simulink model "reshapedevel"  (Simulink 7.4)
settings: Solver=ode45  StartTime=0.0  StopTime=800  RelTol=1e-3
libraries: xbsIndex_r4 x41, casper_library_misc x3
settings Model: Creator=gjones  LastModifiedBy=gjones

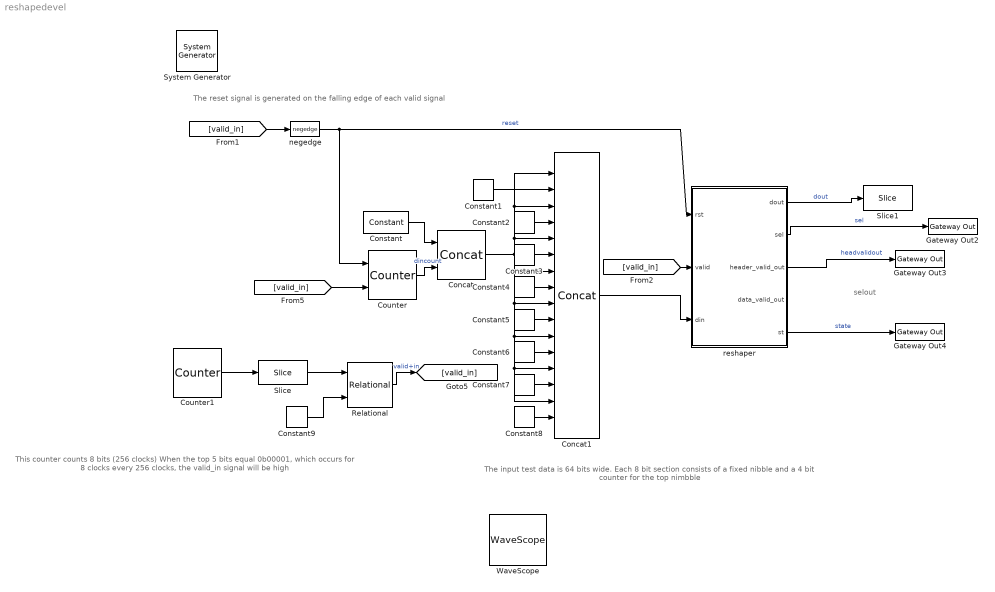
== system reshapedevel ==
  note: selout
  note: This counter counts 8 bits (256 clocks)
      | When the top 5 bits equal 0b00001, which occurs for 8
      | clocks every 256 clocks, the valid_in signal will be high
  note: The reset signal is generated on the falling edge of each valid signal
  note: The input test data is 64 bits wide. Each 8 bit section consists of a fixed nibble and
      |  a 4 bit counter for the top nimbble
  " System Generator" : xbsIndex_r4/ System Generator  Tag=genX  SystemSampleTime=-1  xilinxfamily=Virtex6  part=xc6vsx315t  speed=-3  package=ff1156  synthesis_tool=XST  clock_wrapper=Clock Enables  directory=./netlist  testbench=off  simulink_period=1  sysclk_period=10  dcm_input_clock_period=10  incr_netlist=off  trim_vbits=Everywhere in SubSystem  dbl_ovrd=According to Block Masks  core_generation=According to Block Masks  run_coregen=off  deprecated_control=off  eval_field=0  block_type=sysgen
      settings: block_version=11.4
  Concat : xbsIndex_r4/Concat  num_inputs=2  dbl_ovrd=off  block_type=concat
  Concat1 : xbsIndex_r4/Concat  num_inputs=16  dbl_ovrd=off  block_type=concat
  Constant : xbsIndex_r4/Constant  arith_type=Unsigned  const=0  n_bits=1  bin_pt=0  explicit_period=on  period=1  equ=P=C  opselect=C  inp2=PCIN>>17  opr=+  inp1=P  carry=CIN  dbl_ovrd=off  block_type=constant
      settings: block_version=11.4
  Constant1 : xbsIndex_r4/Constant  arith_type=Unsigned  const=0  n_bits=4  bin_pt=0  explicit_period=on  period=1  equ=P=C  opselect=C  inp2=PCIN>>17  opr=+  inp1=P  carry=CIN  dbl_ovrd=off  block_type=constant
      settings: block_version=11.4
  Constant2 : xbsIndex_r4/Constant  arith_type=Unsigned  const=1  n_bits=4  bin_pt=0  explicit_period=on  period=1  equ=P=C  opselect=C  inp2=PCIN>>17  opr=+  inp1=P  carry=CIN  dbl_ovrd=off  block_type=constant
      settings: block_version=11.4
  Constant3 : xbsIndex_r4/Constant  arith_type=Unsigned  const=2  n_bits=4  bin_pt=0  explicit_period=on  period=1  equ=P=C  opselect=C  inp2=PCIN>>17  opr=+  inp1=P  carry=CIN  dbl_ovrd=off  block_type=constant
      settings: block_version=11.4
  Constant4 : xbsIndex_r4/Constant  arith_type=Unsigned  const=3  n_bits=4  bin_pt=0  explicit_period=on  period=1  equ=P=C  opselect=C  inp2=PCIN>>17  opr=+  inp1=P  carry=CIN  dbl_ovrd=off  block_type=constant
      settings: block_version=11.4
  Constant5 : xbsIndex_r4/Constant  arith_type=Unsigned  const=4  n_bits=4  bin_pt=0  explicit_period=on  period=1  equ=P=C  opselect=C  inp2=PCIN>>17  opr=+  inp1=P  carry=CIN  dbl_ovrd=off  block_type=constant
      settings: block_version=11.4
  Constant6 : xbsIndex_r4/Constant  arith_type=Unsigned  const=5  n_bits=4  bin_pt=0  explicit_period=on  period=1  equ=P=C  opselect=C  inp2=PCIN>>17  opr=+  inp1=P  carry=CIN  dbl_ovrd=off  block_type=constant
      settings: block_version=11.4
  Constant7 : xbsIndex_r4/Constant  arith_type=Unsigned  const=6  n_bits=4  bin_pt=0  explicit_period=on  period=1  equ=P=C  opselect=C  inp2=PCIN>>17  opr=+  inp1=P  carry=CIN  dbl_ovrd=off  block_type=constant
      settings: block_version=11.4
  Constant8 : xbsIndex_r4/Constant  arith_type=Unsigned  const=7  n_bits=4  bin_pt=0  explicit_period=on  period=1  equ=P=C  opselect=C  inp2=PCIN>>17  opr=+  inp1=P  carry=CIN  dbl_ovrd=off  block_type=constant
      settings: block_version=11.4
  Constant9 : xbsIndex_r4/Constant  arith_type=Unsigned  const=1  n_bits=4  bin_pt=0  explicit_period=on  period=1  equ=P=C  opselect=C  inp2=PCIN>>17  opr=+  inp1=P  carry=CIN  dbl_ovrd=off  block_type=constant
      settings: block_version=11.4
  Counter : xbsIndex_r4/Counter  cnt_type=Free Running  cnt_to=Inf  operation=Up  start_count=0  cnt_by_val=1  arith_type=Unsigned  n_bits=3  bin_pt=0  load_pin=off  rst=on  en=on  explicit_period=on  period=1  dbl_ovrd=off  use_behavioral_HDL=off  implementation=Fabric  block_type=counter
      settings: block_version=11.4
  Counter1 : xbsIndex_r4/Counter  cnt_type=Free Running  cnt_to=Inf  operation=Up  start_count=0  cnt_by_val=1  arith_type=Unsigned  n_bits=8  bin_pt=0  load_pin=off  rst=off  en=off  explicit_period=on  period=1  dbl_ovrd=off  use_behavioral_HDL=off  implementation=Fabric  block_type=counter
      settings: block_version=11.4
  Gateway Out2 : xbsIndex_r4/Gateway Out  hdl_port=on  timing_constraint=None  locs_specified=off  LOCs={}  block_type=gatewayout
      settings: infoedit="Gateway out block.  Converts Xilinx fixed point inputs into ouputs of type Simulink integer, double, or fixed point.<br><br>Hardware notes:  In hardware these blocks become top level output ports or are discarded, depending on how they are configured."  block_version=11.4
  Gateway Out3 : xbsIndex_r4/Gateway Out  hdl_port=on  timing_constraint=None  locs_specified=off  LOCs={}  block_type=gatewayout
      settings: infoedit="Gateway out block.  Converts Xilinx fixed point inputs into ouputs of type Simulink integer, double, or fixed point.<br><br>Hardware notes:  In hardware these blocks become top level output ports or are discarded, depending on how they are configured."  block_version=11.4
  Gateway Out4 : xbsIndex_r4/Gateway Out  hdl_port=on  timing_constraint=None  locs_specified=off  LOCs={}  block_type=gatewayout
      settings: infoedit="Gateway out block.  Converts Xilinx fixed point inputs into ouputs of type Simulink integer, double, or fixed point.<br><br>Hardware notes:  In hardware these blocks become top level output ports or are discarded, depending on how they are configured."  block_version=11.4
  Relational : xbsIndex_r4/Relational  mode=a=b  en=off  latency=0  dbl_ovrd=off  block_type=relational
  Slice : xbsIndex_r4/Slice  nbits=5  boolean_output=off  mode=Upper Bit Location + Width  bit1=0  base1=MSB of Input  bit0=0  base0=LSB of Input  dbl_ovrd=off  block_type=slice
  Slice1 : xbsIndex_r4/Slice  nbits=4  boolean_output=off  mode=Upper Bit Location + Width  bit1=0  base1=MSB of Input  bit0=0  base0=LSB of Input  dbl_ovrd=off  block_type=slice
  WaveScope : xbsIndex_r4/WaveScope  block_type=wavescope
      settings: block_version=11.4
  negedge : casper_library_misc/negedge  Tag=Rising Edge Detector  SystemSampleTime=-1
  reshaper : Subsystem  mask{inwid=64, inlen=8, outwid=8, outchunk=16, headlen=11}
      mask prompts: inwid "Input Width (bits)"; inlen "Input Length (clocks)"; outwid "Output Width (bits)"; outchunk "Output Chunk Length (clocks)"; headlen "Header Length"
      mask help:
      | This block takes wide input data and reshapes it to a narrower (or the same)
      | bit width, and breaks it into packets, between which a header can be inserted.
      | Each input data frame must be proceeded by a reset pulse. The input data can be
      | disjoint, with a pulsed valid signal. When the reset signal is pulsed, the previous data
      | frame will be read out. Therefore the number of clocks to read out the header and
      | data must be greater than the number of clocks between two frames (rst signals).
      |
      | The sel signal can be used to drive the select input of a mux which muxes between
      | the data stream (dout) and the indicated number of header words. The header_valid_out
      | signal goes high for each word of the header. dout should be connected to input
      | 0 of the mux. The data_valid_out goes high for each output data value. The st output
      | is for debug access to the internal state machine state.
      mask init:
      | l2inlen = ceil(log2(inlen))
      | l2outchunk = ceil(log2(outchunk))
      | outlen = inlen*(inwid/outwid)
      | nchunk = outlen/outchunk
      | l2headlen = ceil(log2(headlen))
      | l2outlen = ceil(log2(outlen))
  wires:
  Constant/1 -> Concat/1
  Counter/1 -> Concat/2  "dincount"
  Concat/1 -> Concat1/1, Concat1/3, Concat1/5, Concat1/7, Concat1/9, Concat1/11, Concat1/13, Concat1/15
  Constant1/1 -> Concat1/2
  Constant2/1 -> Concat1/4
  Constant3/1 -> Concat1/6
  Constant4/1 -> Concat1/8
  Constant5/1 -> Concat1/10
  Constant6/1 -> Concat1/12
  Constant7/1 -> Concat1/14
  Constant8/1 -> Concat1/16
  Concat1/1 -> reshaper/3(din)
  negedge/1 -> Counter/1, reshaper/1(rst)  "reset"
  Counter1/1 -> Slice/1
  Slice/1 -> Relational/1
  Constant9/1 -> Relational/2
  Relational/1 -> [valid_in]  "valid+in"
  reshaper/1(dout) -> Slice1/1  "dout"
  reshaper/2(sel) -> Gateway Out2/1  "sel"
  reshaper/3(header_valid_out) -> Gateway Out3/1  "headvalidout"
  reshaper/5(st) -> Gateway Out4/1  "state"
  [valid_in] -> Counter/2
  [valid_in] -> negedge/1
  [valid_in] -> reshaper/2(valid)

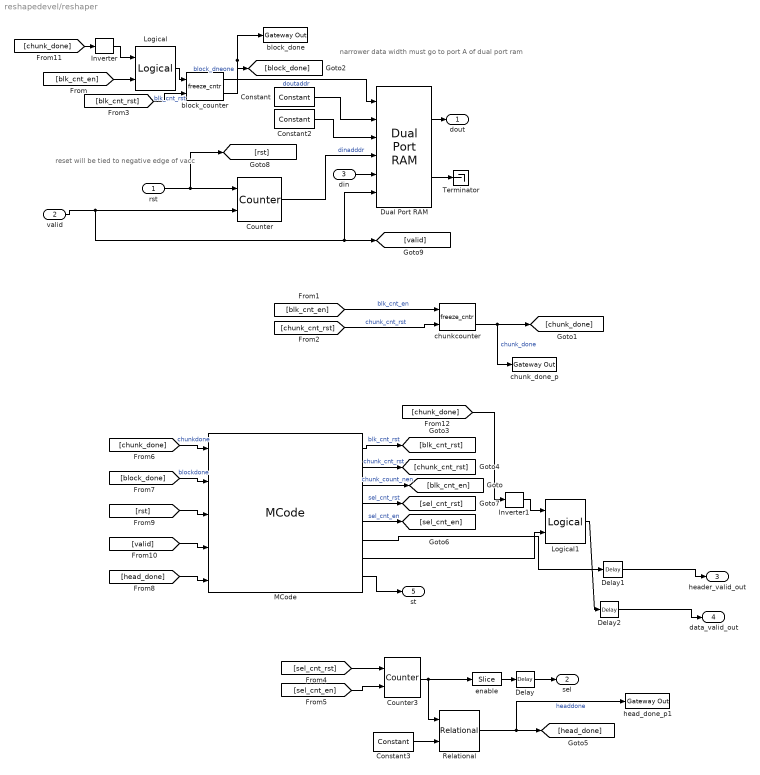
== system reshapedevel/reshaper ==
  note: narrower data width must go to port A of dual port ram
  note: reset will be tied to negative edge
      | of vacc
  rst : Inport
  valid : Inport  Port=2
  din : Inport  Port=3
  Constant : xbsIndex_r4/Constant  arith_type=Unsigned  const=0  n_bits=outwid  bin_pt=0  explicit_period=on  period=1  equ=P=C  opselect=C  inp2=PCIN>>17  opr=+  inp1=P  carry=CIN  dbl_ovrd=off  block_type=constant
      settings: block_version=11.4
  Constant2 : xbsIndex_r4/Constant  arith_type=Boolean  const=0  n_bits=outwid  bin_pt=0  explicit_period=on  period=1  equ=P=C  opselect=C  inp2=PCIN>>17  opr=+  inp1=P  carry=CIN  dbl_ovrd=off  block_type=constant
      settings: block_version=11.4
  Constant3 : xbsIndex_r4/Constant  arith_type=Unsigned  const=headlen  n_bits=l2headlen  bin_pt=0  explicit_period=on  period=1  equ=P=C  opselect=C  inp2=PCIN>>17  opr=+  inp1=P  carry=CIN  dbl_ovrd=off  block_type=constant
      settings: block_version=11.4
  Counter : xbsIndex_r4/Counter  cnt_type=Free Running  cnt_to=Inf  operation=Up  start_count=0  cnt_by_val=1  arith_type=Unsigned  n_bits=l2inlen  bin_pt=0  load_pin=off  rst=on  en=on  explicit_period=on  period=1  dbl_ovrd=off  use_behavioral_HDL=off  implementation=Fabric  block_type=counter
      settings: block_version=11.4
  Counter3 : xbsIndex_r4/Counter  cnt_type=Free Running  cnt_to=1023  operation=Up  start_count=0  cnt_by_val=1  arith_type=Unsigned  n_bits=l2headlen + 1  bin_pt=0  load_pin=off  rst=on  en=on  explicit_period=on  period=1  dbl_ovrd=off  use_behavioral_HDL=off  implementation=Fabric  use_rpm=on  block_type=counter
      settings: xl_area=[0, 0, 0, 0, 0, 0, 0]  block_version=9.1.01
  Delay : xbsIndex_r4/Delay  en=off  latency=1  dbl_ovrd=off  reg_retiming=off  block_type=delay
      settings: block_version=11.4
  Delay1 : xbsIndex_r4/Delay  en=off  latency=2  dbl_ovrd=off  reg_retiming=off  block_type=delay
      settings: block_version=11.4
  Delay2 : xbsIndex_r4/Delay  en=off  latency=2  dbl_ovrd=off  reg_retiming=off  block_type=delay
      settings: block_version=11.4
  Dual Port RAM : xbsIndex_r4/Dual Port RAM  depth=outlen  initVector=sin(pi*(0:outlen)/16)  distributed_mem=Block RAM  init_a=0  init_b=0  rst_a=off  rst_b=off  en_a=off  en_b=off  latency=2  write_mode_A=Read After Write  write_mode_B=Read After Write  dbl_ovrd=off  optimize=Speed  use_rpm=on  block_type=dpram
      settings: block_version=11.4
  Inverter : xbsIndex_r4/Inverter  en=off  latency=0  dbl_ovrd=off  block_type=inv
      settings: block_version=11.4
  Inverter1 : xbsIndex_r4/Inverter  en=off  latency=0  dbl_ovrd=off  block_type=inv
      settings: block_version=11.4
  Logical : xbsIndex_r4/Logical  logical_function=AND  inputs=2  en=off  latency=0  precision=Full  arith_type=Unsigned  n_bits=16  bin_pt=0  align_bp=on  dbl_ovrd=off  block_type=logical
      settings: block_version=11.4
  Logical1 : xbsIndex_r4/Logical  logical_function=AND  inputs=2  en=off  latency=0  precision=Full  arith_type=Unsigned  n_bits=16  bin_pt=0  align_bp=on  dbl_ovrd=off  block_type=logical
      settings: block_version=11.4
  MCode : xbsIndex_r4/MCode  mfname=reshaper_fsm.m  explicit_period=off  period=1  inputsTable={'boundInpExpr'=>['','','','',''],'inputs'=>['end_chunk','end_block','rst','valid_in','head_done']}  outputsTable={'outputs'=>['block_count_rst','chunk_count_rst','chunk_count_en','sel_rst','sel_en','header_valid','data_valid','st'],'suppressOut'=>['off','off','off','off','off','off','off','off']}  dbl_ovrd=off  enable_stdout=off  enable_debug=off  suppress_output=on  defparams={}  hide_port_list={}  block_type=mcode
      settings: block_version=11.4
  Relational : xbsIndex_r4/Relational  mode=a>=b  en=off  latency=0  dbl_ovrd=off  block_type=relational
  Terminator : Terminator
  block_counter : casper_library_misc/freeze_cntr  SystemSampleTime=-1  CounterBits=l2outlen
  block_done : xbsIndex_r4/Gateway Out  hdl_port=off  timing_constraint=None  locs_specified=off  LOCs={}  block_type=gatewayout
      settings: infoedit="Gateway out block.  Converts Xilinx fixed point inputs into ouputs of type Simulink integer, double, or fixed point.<br><br>Hardware notes:  In hardware these blocks become top level output ports or are discarded, depending on how they are configured."  block_version=11.4
  chunk_done_p : xbsIndex_r4/Gateway Out  hdl_port=off  timing_constraint=None  locs_specified=off  LOCs={}  block_type=gatewayout
      settings: infoedit="Gateway out block.  Converts Xilinx fixed point inputs into ouputs of type Simulink integer, double, or fixed point.<br><br>Hardware notes:  In hardware these blocks become top level output ports or are discarded, depending on how they are configured."  block_version=11.4
  chunkcounter : casper_library_misc/freeze_cntr  SystemSampleTime=-1  CounterBits=l2outchunk
  enable : xbsIndex_r4/Slice  nbits=l2headlen  boolean_output=off  mode=Lower Bit Location + Width  bit1=0  base1=LSB of Input  bit0=0  base0=LSB of Input  dbl_ovrd=off  block_type=slice
      settings: block_version=9.1.01
  head_done_p1 : xbsIndex_r4/Gateway Out  hdl_port=off  timing_constraint=None  locs_specified=off  LOCs={}  block_type=gatewayout
      settings: infoedit="Gateway out block.  Converts Xilinx fixed point inputs into ouputs of type Simulink integer, double, or fixed point.<br><br>Hardware notes:  In hardware these blocks become top level output ports or are discarded, depending on how they are configured."  block_version=11.4
  dout : Outport
  sel : Outport  Port=2
  header_valid_out : Outport  Port=3
  data_valid_out : Outport  Port=4
  st : Outport  Port=5
  wires:
  rst/1 -> Counter/1, [rst]
  valid/1 -> Counter/2, [valid], Dual Port RAM/6
  [blk_cnt_en] -> chunkcounter/1  "blk_cnt_en"
  chunkcounter/3 -> [chunk_done], chunk_done_p/1  "chunk_done"
  [chunk_cnt_rst] -> chunkcounter/2  "chunk_cnt_rst"
  block_counter/3 -> [block_done], block_done/1  "block_dneone"
  [blk_cnt_rst] -> block_counter/2  "blk_cnt_rst"
  MCode/3 -> [blk_cnt_en]  "chunk_count_nen"
  MCode/1 -> [blk_cnt_rst]  "blk_cnt_rst"
  MCode/2 -> [chunk_cnt_rst]  "chunk_cnt_rst"
  [sel_cnt_rst] -> Counter3/1
  Counter3/1 -> enable/1, Relational/1
  Constant3/1 -> Relational/2
  [sel_cnt_en] -> Counter3/2
  enable/1 -> Delay/1
  Relational/1 -> [head_done], head_done_p1/1  "headdone"
  MCode/5 -> [sel_cnt_en]  "sel_cnt_en"
  MCode/4 -> [sel_cnt_rst]  "sel_cnt_rst"
  [chunk_done] -> MCode/1  "chunkdone"
  [block_done] -> MCode/2  "blockdone"
  [head_done] -> MCode/5
  [rst] -> MCode/3
  [valid] -> MCode/4
  Dual Port RAM/1 -> dout/1
  Dual Port RAM/2 -> Terminator/1
  block_counter/1 -> Dual Port RAM/1  "doutaddr"
  Constant/1 -> Dual Port RAM/2
  Constant2/1 -> Dual Port RAM/3
  Counter/1 -> Dual Port RAM/4  "dinadddr"
  din/1 -> Dual Port RAM/5
  Delay/1 -> sel/1
  Delay1/1 -> header_valid_out/1
  [blk_cnt_en] -> Logical/2
  Logical/1 -> block_counter/1
  Inverter/1 -> Logical/1
  [chunk_done] -> Inverter/1
  Inverter1/1 -> Logical1/1
  [chunk_done] -> Inverter1/1
  MCode/8 -> st/1
  MCode/6 -> Delay1/1
  Delay2/1 -> data_valid_out/1
  MCode/7 -> Logical1/2
  Logical1/1 -> Delay2/1
